simulink model "dronedp"  (R2024b)
settings: Solver=VariableStepAuto  StartTime=0.0  StopTime=10.0  RelTol=1e-3
libraries: vrlib x1
settings Model: LastModifiedBy=Mani_Reddy

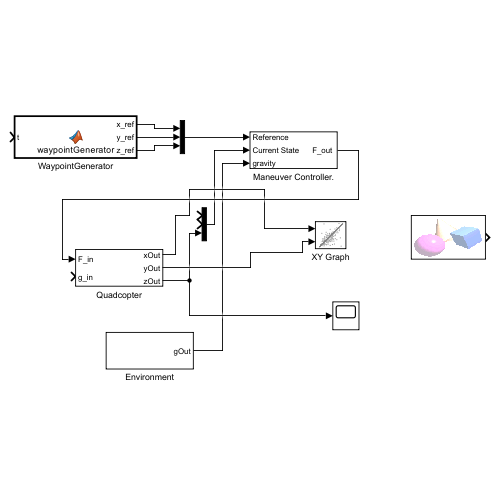
[thumbnail: Simulink's stored preview of the top-level diagram]
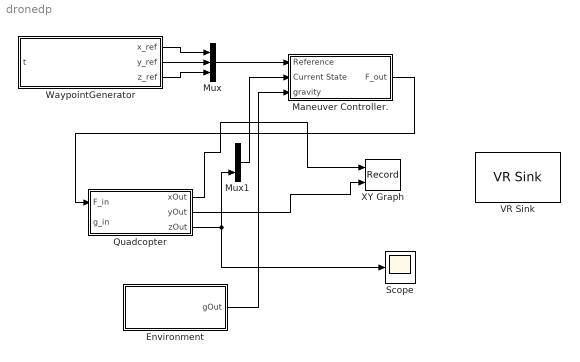
== system dronedp ==
  Environment : Subsystem
  Maneuver Controller. : Subsystem
  Mux : Mux  Inputs=3
  Mux1 : Mux  Inputs=3
  Quadcopter : Subsystem
  Scope : Scope
  VR Sink : vrlib/VR Sink  InstantiateOnLoad=on  SampleTime=0.1  ViewEnable=on  RemoteChange=off  RemoteView=off  WorldFileName=drone 3d\drone.wrl  AutoView=off  VideoDimensions=[200 320]  AllowVariableSize=off  FigureProperties="{'Position', 'Name', 'Viewpoint', 'CameraBound', 'CameraDirection', 'CameraPosition', 'CameraUpVector', 'ZoomFactor', 'Antialiasing', 'Headlight', 'Lighting', 'Sound', 'StatusBar', 'Stereo3D', 'Stereo3DCameraOffset', 'Stereo3DHIT', 'ToolBar', 'Textures', 'Transparency', 'Triad', 'Wireframe', 'NavZones', 'NavMode', 'NavSpeed', 'CaptureFileFormat', 'CaptureFileName', 'Record2DCompressMethod', 'Record2DCompressQuality', 'Record2D', 'Record2DFileName', 'Record2DFPS', 'NavPanel'; [5.0000000000000000e+00   6.0000000000000000e+01   2.5600000000000000e+02   1.6000000000000000e+02], '', '', 'on', [6.0821951424396892e-02   1.2530243358856186e-01   9.9025248818759182e-01], [-7.0135738673040535e+01   7.4789479536459808e+01  -5.5391740588903633e+02], [-7.6875512221906087e-03   9.9211859175339412e-01  -1.2506638818431076e-01], [1.0000000000000000e+00], 'on', 'on', 'on', 'on', 'off', 'off', [1.0000000149011612e-01], [0.0000000000000000e+00], 'off', 'on', 'on', 'none', 'off', 'off', 'fly', 'normal', 'tif', '%f_anim_%n.tif', 'auto', [7.5000000000000000e+01], 'off', '***video***', 'auto', 'none'}"
  WaypointGenerator : MATLAB Function  TreatAsAtomicUnit=on
  XY Graph : Record  FileSettingsInternal="{\"entries\":[{\"content\":{\"excelSettings\":{\"content\":{},\"type\":\"Streamout.ExcelSettings\"}},\"type\":\"Streamout.FileSettingStorage\",\"uuid\":\"\"}],\"packageUris\":[\"http:\\/\\/schema.mathworks.com\\/mf0\\/streamout_blocks\\/R2020a\"],\"version\":\"1.0\"}"  Layout=[1 1]  SignalsInternal="{\"entries\":[{\"content\":{\"signals\":[{\"content\":{\"blockPath\":[],\"dimensions\":[1],\"domain\":\"\",\"lineColor\":\"#a2142f\",\"plots\":[ 1 ],\"port\":1,\"signalID\":1,\"signalName\":\"Quadcopter:1\"},\"type\":\"RecordBlkView.Signal\",\"uuid\":\"\"},{\"content\":{\"blockPath\":[],\"dimensions\":[1],\"domain\":\"\",\"lineColor\":\"#139fff\",\"plots\":[ 1 ],\"port\":2,\"signalID\":2,\"signalName\":\"Quadcopter:2\"},\"type\":\"RecordBlkView.Signal\",\"uuid\":\"\"}]},\"type\":\"RecordBlkView.InputSignals\",\"uuid\":\"\"}],\"packageUris\":[\"http:\\/\\/schema.mathworks.com\\/mf0\\/streamout_blocks\\/R2020a\"],\"version\":\"1.0\"}"  VisualizationBindings="{\"xyplotplugin\":{\"info\":[{\"series\":[{\"bindingParametersList\":[{\"parameter\":\"X-Axis\",\"signalID\":1,\"signalName\":\"Quadcopter:1\"},{\"parameter\":\"Y-Axis\",\"signalID\":2,\"signalName\":\"Quadcopter:2\"}],\"seriesID\":0}],\"subplotID\":1}]}}"  CompatibilityTag=XY
  wires:
  Maneuver Controller./1("F_out ") -> Quadcopter/1(F_in)
  WaypointGenerator/1(x_ref) -> Mux/1
  WaypointGenerator/2(y_ref) -> Mux/2
  WaypointGenerator/3(z_ref) -> Mux/3
  Mux/1 -> Maneuver Controller./1(Reference)
  Environment/1(gOut) -> Maneuver Controller./3(gravity)
  Quadcopter/1(xOut) -> XY Graph/1
  Quadcopter/2(yOut) -> XY Graph/2
  Quadcopter/3(zOut) -> Scope/1, Mux1/3
  Mux1/1 -> Maneuver Controller./2(Current State)

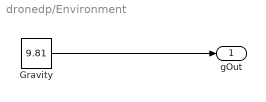
== system dronedp/Environment ==
  Gravity : Constant  Value=9.81
  gOut : Outport
  wires:
  Gravity/1 -> gOut/1

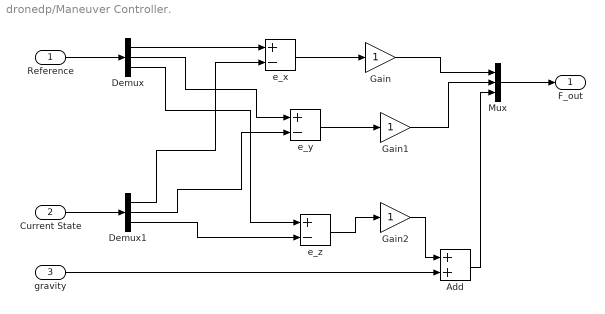
== system dronedp/Maneuver Controller. ==
  Reference : Inport
  Current State : Inport  Port=2
  gravity : Inport  Port=3
  Add : Sum
  Demux : Demux  Outputs=3
  Demux1 : Demux  Outputs=3
  Gain : Gain
  Gain1 : Gain
  Gain2 : Gain
  Mux : Mux  Inputs=3
  e_x : Sum  Inputs=+-
  e_y : Sum  Inputs=+-
  e_z : Sum  Inputs=+-
  "F_out " : Outport
  wires:
  e_x/1 -> Gain/1
  e_y/1 -> Gain1/1
  e_z/1 -> Gain2/1
  Gain2/1 -> Add/1
  Gain/1 -> Mux/1
  Gain1/1 -> Mux/2
  Add/1 -> Mux/3
  Mux/1 -> "F_out "/1
  gravity/1 -> Add/2
  Reference/1 -> Demux/1
  Demux/1 -> e_x/1
  Demux/2 -> e_y/1
  Demux/3 -> e_z/1
  Current State/1 -> Demux1/1
  Demux1/1 -> e_x/2
  Demux1/2 -> e_y/2
  Demux1/3 -> e_z/2

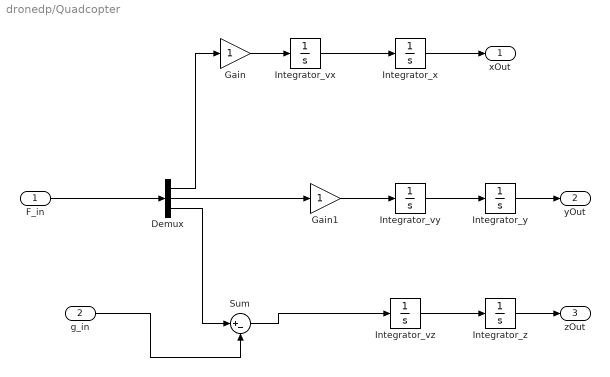
== system dronedp/Quadcopter ==
  F_in : Inport
  g_in : Inport  Port=2
  Demux : Demux  Outputs=3
  Gain : Gain
  Gain1 : Gain
  Integrator_vx : Integrator
  Integrator_vy : Integrator
  Integrator_vz : Integrator
  Integrator_x : Integrator
  Integrator_y : Integrator
  Integrator_z : Integrator
  Sum : Sum  Inputs=|+-
  xOut : Outport
  yOut : Outport  Port=2
  zOut : Outport  Port=3
  wires:
  F_in/1 -> Demux/1
  Demux/1 -> Gain/1
  Gain/1 -> Integrator_vx/1
  Integrator_vx/1 -> Integrator_x/1
  Integrator_x/1 -> xOut/1
  Demux/2 -> Gain1/1
  Gain1/1 -> Integrator_vy/1
  Integrator_vy/1 -> Integrator_y/1
  Integrator_y/1 -> yOut/1
  Demux/3 -> Sum/1
  g_in/1 -> Sum/2
  Sum/1 -> Integrator_vz/1
  Integrator_vz/1 -> Integrator_z/1
  Integrator_z/1 -> zOut/1

== matlab function dronedp/WaypointGenerator ==
  data: t input; x_ref output; y_ref output; z_ref output
function [x_ref, y_ref, z_ref] = waypointGenerator(t)
% This function outputs (x_ref, y_ref, z_ref) as the drone reference.
% The drone will move between waypoints in a piecewise-linear fashion.

% 1) Define your waypoints (x, y, z). You can add or remove as needed.
persistent waypoints
if isempty(waypoints)
    waypoints = [
        0   0   0;  % Start
        5   0   0;  % Move 5m in X
        5   5   0;  % Then 5m in Y
        5   5   5;  % Then go up in Z
        0   5   5;  
        0   0   5;  
        0   0   0   % Return to start
    ];
end

% 2) Time to move between each pair of waypoints
segmentTime = 2;  % seconds per segment

% 3) Calculate how many segments
numSegments = size(waypoints,1) - 1;  
totalTime = numSegments * segmentTime;

% If time > totalTime, stay at final waypoint
if t >= totalTime
    x_ref = waypoints(end,1);
    y_ref = waypoints(end,2);
    z_ref = waypoints(end,3);
    return;
end

% Determine which segment we're in (1-based)
currentSegment = floor(t / segmentTime) + 1;  
% Time inside the current segment
localT = mod(t, segmentTime);

% Start and end points of this segment
startWP = waypoints(currentSegment, :);
endWP   = waypoints(currentSegment+1, :);

% Interpolation factor from 0 to 1
alpha = localT / segmentTime;

% Linear interpolation for x, y, z
x_ref = (1-alpha)*startWP(1) + alpha*endWP(1);
y_ref = (1-alpha)*startWP(2) + alpha*endWP(2);
z_ref = (1-alpha)*startWP(3) + alpha*endWP(3);
end
